simulink model "LQG_tw_v2"  (R2019a)
settings: Solver=FixedStepAuto  StartTime=0.0  StopTime=15  FixedStep=0.01  RelTol=1e-3
undefined symbols (not defined in the file): AA, BB, C, K, L
libraries: simulink x2, simulink_extras x1
settings Model: Creator=chute  LastModifiedBy=chute
settings DataIOCC: ReturnWorkspaceOutputs=off

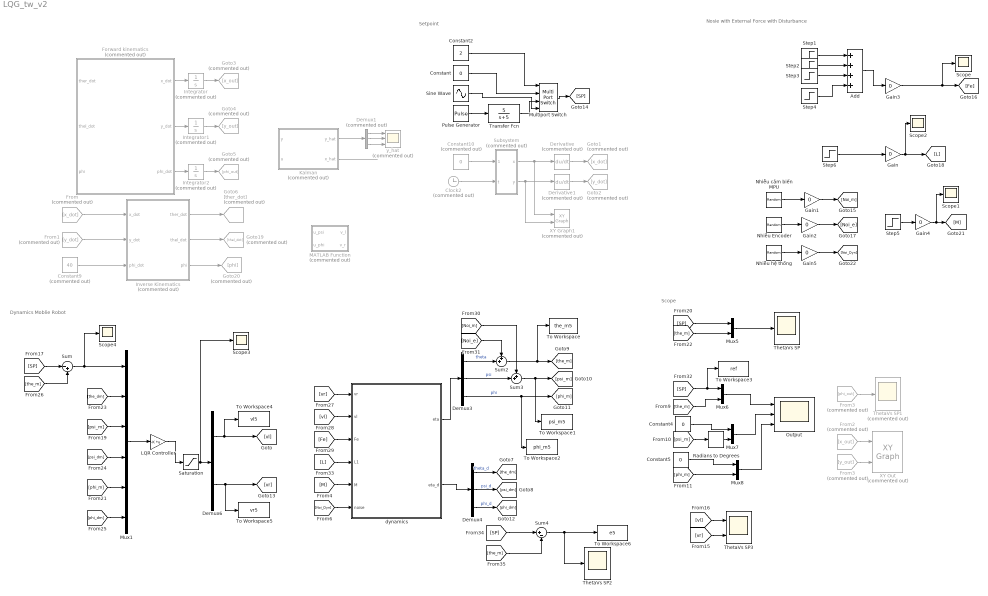
== system LQG_tw_v2 ==
  note: Nosie with External Force with Disturbance
  note: Scope
  note: Setpoint
  note: Dynamics Moblie Robot
  Add : Sum  Inputs=++++
  Clock2 : Clock  Commented=on
  Constant : Constant  Value=0
  Constant10 : Constant  Commented=on  Value=0
  Constant2 : Constant  Value=2
  Constant4 : Constant  Value=0
  Constant5 : Constant  Value=0
  Constant9 : Constant  Commented=on  Value=40
  Demux1 : Demux  Commented=on  Outputs=3
  Demux3 : Demux  Outputs=3
  Demux4 : Demux  Outputs=3
  Demux6 : Demux  Outputs=2
  Derivative : Derivative  Commented=on
  Derivative1 : Derivative  Commented=on
  Forward kinematics : MATLAB Function  Commented=on  TreatAsAtomicUnit=on
  From : From  Commented=on  GotoTag=x_dot
  From1 : From  Commented=on  GotoTag=y_dot
  From2 : From  Commented=on  GotoTag=x_out
  From3 : From  Commented=on  GotoTag=phi_out
  "From3 " : From  Commented=on  GotoTag=y_out
  Gain{,1..5} (6 alike) : Gain  Gain=0
  Goto1 : Goto  Commented=on  GotoTag=x_dot
  Goto19 : Goto  Commented=on  GotoTag=thel_dot
  Goto2 : Goto  Commented=on  GotoTag=y_dot
  Goto20 : Goto  Commented=on  GotoTag=phi
  Goto3 : Goto  Commented=on  GotoTag=x_out
  Goto4 : Goto  Commented=on  GotoTag=y_out
  Goto5 : Goto  Commented=on  GotoTag=phi_out
  Goto6 : Goto  Commented=on  GotoTag=ther_dot
  Integrator : Integrator  Commented=on
  Integrator1 : Integrator  Commented=on
  Integrator2 : Integrator  Commented=on  InitialCondition=[0;0]
  Inverse Kinematics : MATLAB Function  Commented=on  TreatAsAtomicUnit=on
  Kalman : Subsystem  Commented=on
  LQR Controller : Gain  Gain=-K  Multiplication=Matrix(K*u) (u vector)
  MATLAB Function : MATLAB Function  Commented=on  TreatAsAtomicUnit=on
  Multiport Switch : MultiPortSwitch
  Mux1 : Mux  Inputs=6
  Mux{5..8} (4 alike) : Mux  Inputs=2
  Nhiễu Encoder : RandomNumber  Variance=0.0001  SampleTime=0.01
  Nhiễu cảm biến MPU : RandomNumber  Variance=0.0005  SampleTime=0.01
  Nhiễu hệ thống : RandomNumber  Variance=0.0001  SampleTime=0.01
  Output : Scope  NumInputPorts=3
  Pulse Generator : DiscretePulseGenerator  PulseType=Time based  Amplitude=3.14  Period=10  PulseWidth=50
  Radians to Degrees : simulink_extras/Transformations/Radians to Degrees
  Saturation : Saturate  UpperLimit=12  LowerLimit=-12
  Scope{,1..4} (5 alike) : Scope
  Sine Wave : Sin  Amplitude=3.14  Frequency=0.1*pi  SampleTime=0
  Step1 : Step  Time=3  After=0.3  SampleTime=0
  Step2 : Step  Time=4  After=-0.3  SampleTime=0
  Step3 : Step  Time=10  After=0.3  SampleTime=0
  Step4 : Step  Time=11  After=-0.3  SampleTime=0
  Step5 : Step  Time=8  Before=0.945  After=1000  SampleTime=0
  Step6 : Step  Time=5  Before=0.121/2  After=0.121/2+0.1  SampleTime=0
  Subsystem : Subsystem  Commented=on
  Sum : Sum  Inputs=|-+
  Sum2 : Sum  Inputs=++|
  Sum3 : Sum  Inputs=++|
  Sum4 : Sum  Inputs=|+-
  ThetaVs SP : Scope
  ThetaVs SP1 : Scope  Commented=on
  ThetaVs SP2 : Scope
  ThetaVs SP3 : Scope  NumInputPorts=2
  To Workspace : ToWorkspace  VariableName=the_m5  SaveFormat=Structure With Time  SampleTime=-1
  To Workspace1 : ToWorkspace  VariableName=psi_m5  SaveFormat=Structure With Time  SampleTime=-1
  To Workspace2 : ToWorkspace  VariableName=phi_m5  SaveFormat=Structure With Time  SampleTime=-1
  To Workspace3 : ToWorkspace  VariableName=ref  SaveFormat=Structure With Time  SampleTime=-1
  To Workspace4 : ToWorkspace  VariableName=vl5  SaveFormat=Structure With Time  SampleTime=-1
  To Workspace5 : ToWorkspace  VariableName=vr5  SaveFormat=Structure With Time  SampleTime=-1
  To Workspace6 : ToWorkspace  VariableName=e5  SaveFormat=Structure With Time  SampleTime=-1
  Transfer Fcn : TransferFcn  Numerator=[5]  Denominator="[1  5]"
  XY Graph1 : simulink/Sinks/XY Graph  Commented=on  xmin=-1  xmax=1  ymin=-1  ymax=1  st=-1
  XY Out : simulink/Sinks/XY Graph  Commented=on  xmin=-1  xmax=1  ymin=-1  ymax=1  st=-1
  dynamics : Subsystem
  y_hat : Scope  Commented=on  NumInputPorts=3
  wires:
  dynamics/1(eta) -> Demux3/1
  Demux4/1 -> [the_dm]  "theta_d"
  dynamics/2(eta_d) -> Demux4/1
  Demux4/3 -> [phi_dm]  "phi_d"
  Demux4/2 -> [psi_dm]  "psi_d"
  Demux6/1 -> To Workspace4/1, [vl]
  LQR Controller/1 -> Saturation/1
  Mux1/1 -> LQR Controller/1
  Sum/1 -> Scope4/1, Mux1/1
  Multiport Switch/1 -> [SP]
  Constant/1 -> Multiport Switch/2
  Constant2/1 -> Multiport Switch/1
  Mux5/1 -> ThetaVs SP/1
  [SP] -> Mux5/1
  [the_m] -> Mux5/2
  [phi_m] -> Mux1/5
  [psi_m] -> Mux1/3
  [the_dm] -> Mux1/2
  [psi_dm] -> Mux1/4
  [phi_dm] -> Mux1/6
  Nhiễu cảm biến MPU/1 -> Gain1/1
  Demux3/3 -> To Workspace2/1, [phi_m]  "phi"
  Sum3/1 -> To Workspace1/1, [psi_m]
  Demux3/2 -> Sum3/2  "psi"
  Demux3/1 -> Sum2/2  "theta"
  Nhiễu Encoder/1 -> Gain2/1
  [the_m] -> Sum/2
  Sine Wave/1 -> Multiport Switch/4
  [vl] -> dynamics/2("vl ")
  [vr] -> dynamics/1(vr)
  [Fe] -> dynamics/3(Fe)
  Gain1/1 -> [Noi_m]
  Gain2/1 -> [Noi_e]
  [Noi_m] -> Sum3/1
  [Noi_e] -> Sum2/1
  Add/1 -> Gain3/1
  Mux8/1 -> Output/3
  Mux7/1 -> Output/2
  Mux6/1 -> Output/1
  [the_m] -> Mux6/2
  [SP] -> To Workspace3/1, Mux6/1
  [psi_m] -> Radians to Degrees/1
  Constant4/1 -> Mux7/1
  [phi_m] -> Mux8/2
  Constant5/1 -> Mux8/1
  [L] -> dynamics/4(L1)
  Step6/1 -> Gain/1
  Gain/1 -> Scope2/1, [L]
  Sum2/1 -> To Workspace/1, [the_m]
  Demux6/2 -> To Workspace5/1, [vr]
  [SP] -> Sum4/1
  [the_m] -> Sum4/2
  Sum4/1 -> ThetaVs SP2/1, To Workspace6/1
  Pulse Generator/1 -> Transfer Fcn/1
  [SP] -> Sum/1
  Transfer Fcn/1 -> Multiport Switch/3
  Forward kinematics/1(x_dot) -> Integrator/1
  Forward kinematics/3(phi_dot) -> Integrator2/1
  Clock2/1 -> Subsystem/2(t)
  Subsystem/1(x) -> Derivative/1, XY Graph1/1
  Constant10/1 -> Subsystem/1(mode)
  Forward kinematics/2(y_dot) -> Integrator1/1
  Constant9/1 -> Inverse Kinematics/3(phi_dot)
  Integrator2/1 -> Goto5/1
  Subsystem/2(y) -> XY Graph1/2, Derivative1/1
  Derivative1/1 -> Goto2/1
  Derivative/1 -> Goto1/1
  From1/1 -> Inverse Kinematics/2(y_dot)
  From/1 -> Inverse Kinematics/1(x_dot)
  Integrator/1 -> Goto3/1
  Integrator1/1 -> Goto4/1
  From2/1 -> XY Out/1
  "From3 "/1 -> XY Out/2
  From3/1 -> ThetaVs SP1/1
  Inverse Kinematics/1(ther_dot) -> Goto6/1
  Inverse Kinematics/2(thel_dot) -> Goto19/1
  Inverse Kinematics/3(phi) -> Goto20/1
  Kalman/1(y_hat) -> Demux1/1
  Demux1/1 -> y_hat/1
  Demux1/3 -> y_hat/3
  Demux1/2 -> y_hat/2
  Kalman/2(x_hat) -> ?
  Step1/1 -> Add/1
  Step2/1 -> Add/2
  Gain3/1 -> Scope/1, [Fe]
  Step4/1 -> Add/4
  Step3/1 -> Add/3
  Step5/1 -> Gain4/1
  Gain4/1 -> Scope1/1, [M]
  [M] -> dynamics/5(M)
  Gain5/1 -> [Noi_Dyn]
  Nhiễu hệ thống/1 -> Gain5/1
  [Noi_Dyn] -> dynamics/6(noise)
  Saturation/1 -> Scope3/1, Demux6/1
  Radians to Degrees/1 -> Mux7/2
  [vl] -> ThetaVs SP3/1
  [vr] -> ThetaVs SP3/2

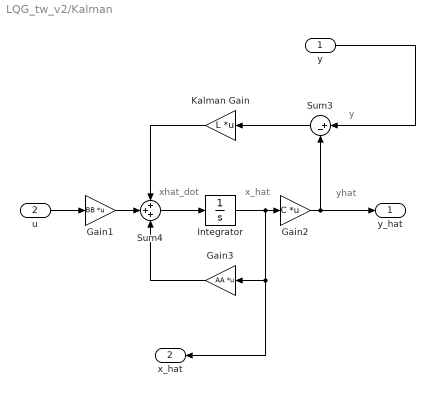
== system LQG_tw_v2/Kalman ==
  note: x_hat
  note: yhat
  note: xhat_dot
  note: y
  y : Inport
  u : Inport  Port=2
  Gain1 : Gain  Gain=BB  Multiplication=Matrix(K*u)
  Gain2 : Gain  Gain=C  Multiplication=Matrix(K*u)
  Gain3 : Gain  Gain=AA  Multiplication=Matrix(K*u)
  Integrator : Integrator  InitialCondition=[0.5;0.01;pi/6;0.001;0.0;0.001]
  Kalman Gain : Gain  Gain=L  Multiplication=Matrix(K*u)
  Sum3 : Sum  Inputs=|+-
  Sum4 : Sum  Inputs=+++
  y_hat : Outport
  x_hat : Outport  Port=2
  wires:
  u/1 -> Gain1/1
  Integrator/1 -> x_hat/1, Gain3/1, Gain2/1
  Gain1/1 -> Sum4/2
  Gain2/1 -> y_hat/1, Sum3/2
  Sum4/1 -> Integrator/1
  y/1 -> Sum3/1
  Gain3/1 -> Sum4/3
  Kalman Gain/1 -> Sum4/1
  Sum3/1 -> Kalman Gain/1

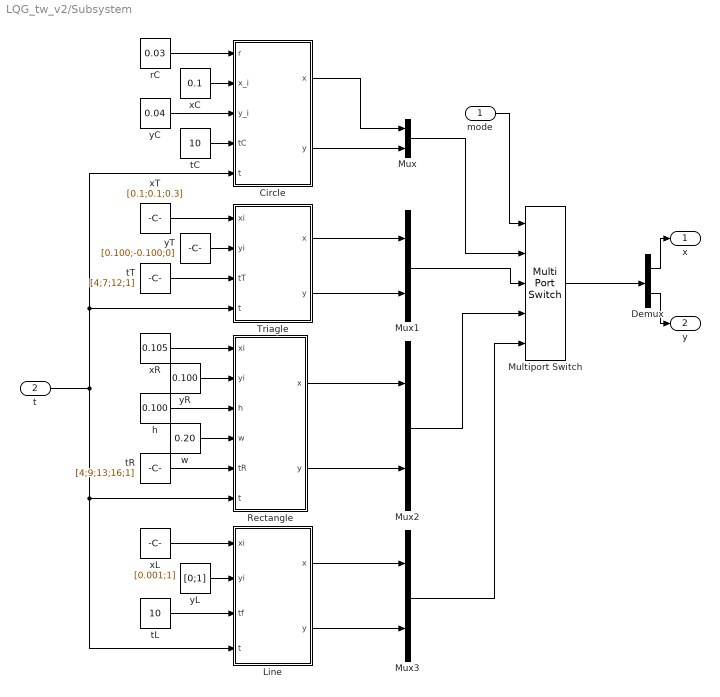
== system LQG_tw_v2/Subsystem ==
  mode : Inport
  t : Inport  Port=2
  Circle : MATLAB Function  TreatAsAtomicUnit=on
  Demux : Demux  Outputs=2
  Line : MATLAB Function  TreatAsAtomicUnit=on
  Multiport Switch : MultiPortSwitch  DataPortOrder=Zero-based contiguous  Inputs=4  zeroidx=on
  Mux{,1..3} (4 alike) : Mux  Inputs=2
  Rectangle : MATLAB Function  TreatAsAtomicUnit=on
  Triagle : MATLAB Function  TreatAsAtomicUnit=on
  h : Constant  Value=0.100
  rC : Constant  Value=0.03
  tC : Constant  Value=10
  tL : Constant  Value=10
  tR : Constant  Value=[4;9;13;16;1]
  tT : Constant  Value=[4;7;12;1]
  w : Constant  Value=0.20
  xC : Constant  Value=0.1
  xL : Constant  Value=[0.001;1]
  xR : Constant  Value=0.105
  xT : Constant  Value=[0.1;0.1;0.3]
  yC : Constant  Value=0.04
  yL : Constant  Value=[0;1]
  yR : Constant  Value=0.100
  yT : Constant  Value=[0.100;-0.100;0]
  x : Outport
  y : Outport  Port=2
  wires:
  tR/1 -> Rectangle/5(tR)
  xL/1 -> Line/1(xi)
  Line/1(x) -> Mux3/1
  tC/1 -> Circle/4(tC)
  yL/1 -> Line/2(yi)
  tT/1 -> Triagle/3(tT)
  Multiport Switch/1 -> Demux/1
  Line/2(y) -> Mux3/2
  Triagle/1(x) -> Mux1/1
  Mux3/1 -> Multiport Switch/5
  xR/1 -> Rectangle/1(xi)
  Circle/2(y) -> Mux/2
  tL/1 -> Line/3(tf)
  w/1 -> Rectangle/4(w)
  Mux2/1 -> Multiport Switch/4
  mode/1 -> Multiport Switch/1
  Circle/1(x) -> Mux/1
  Mux1/1 -> Multiport Switch/3
  rC/1 -> Circle/1(r)
  Mux/1 -> Multiport Switch/2
  h/1 -> Rectangle/3(h)
  t/1 -> Circle/5(t), Triagle/4(t), Rectangle/6(t), Line/4(t)
  Demux/1 -> x/1
  xT/1 -> Triagle/1(xi)
  Rectangle/1(x) -> Mux2/1
  yT/1 -> Triagle/2(yi)
  xC/1 -> Circle/2(x_i)
  Triagle/2(y) -> Mux1/2
  yR/1 -> Rectangle/2(yi)
  Demux/2 -> y/1
  Rectangle/2(y) -> Mux2/2
  yC/1 -> Circle/3(y_i)

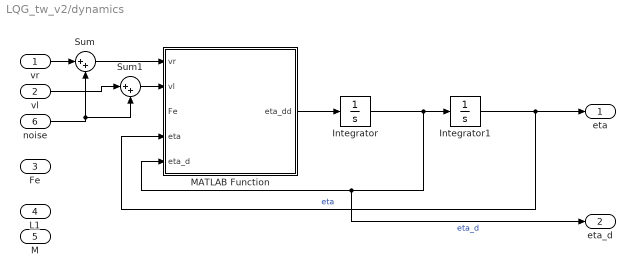
== system LQG_tw_v2/dynamics ==
  vr : Inport
  "vl " : Inport  Port=2
  Fe : Inport  Port=3
  L1 : Inport  Port=4
  M : Inport  Port=5
  noise : Inport  Port=6
  Integrator : Integrator  InitialCondition=[0;0;0]
  Integrator1 : Integrator  InitialCondition=[0;0.3*pi/180;0]
  MATLAB Function : MATLAB Function  TreatAsAtomicUnit=on
  Sum : Sum  Inputs=|++
  Sum1 : Sum  Inputs=|++
  eta : Outport
  eta_d : Outport  Port=2
  wires:
  Integrator/1 -> Integrator1/1, eta_d/1, MATLAB Function/5(eta_d)  "eta_d"
  Integrator1/1 -> eta/1, MATLAB Function/4(eta)  "eta"
  MATLAB Function/1(eta_dd) -> Integrator/1
  vr/1 -> Sum/1
  Sum/1 -> MATLAB Function/1(vr)
  Sum1/1 -> MATLAB Function/2(vl)
  "vl "/1 -> Sum1/1
  noise/1 -> Sum1/2, Sum/2

== matlab function LQG_tw_v2/Forward kinematics ==
  data: ther_dot input; x_dot output; thel_dot input; y_dot output; phi_dot output; phi input
function [x_dot,y_dot,phi_dot] = FK(ther_dot,thel_dot,phi)
R =0.0335; % Wheel radius
W =0.17; % Body width
% thel_dot= (the_dot-(phi_dot*W)/R);
% ther_dot= the_dot+phi_dot*W/(2*R);
for i=1:2
    J=[(R/2)*cos(phi(i)),(R/2)*cos(phi(i));
        (R/2)*sin(phi(i)),(R/2)*sin(phi(i));
        R/W,-R/W];
end
out =J*[ther_dot;thel_dot];
x_dot=out(1,1);
y_dot =out(2,1);
phi_dot =out(3,1);


end

== matlab function LQG_tw_v2/dynamics/MATLAB Function ==
  data: vr input; vl input; Fe input; eta_dd output; eta input; eta_d input
function eta_dd= fcn(vr,vl,Fe,eta,eta_d)
%% declare the parameter:
%% Hoang

g =9.81; % gravity acceleration
m =0.046; % wheel weight
R =0.0335; % Wheel radius
M =0.945;  % body weight
W =0.17; % Body width
D =0.1; % Body depth
H =0.121;% Body Height
L =0.121/2;% distance

n =30 ; %gear ratio
Rm=8.0013;      %dien tro dong co DC
Kb=0.45096;   %he so emf cua dong co
Kt=0.45096;   %momemt xoan cua dong co DC\
fm = 0.21895; % friction cof between body and DC motor.
fw = 0.01; % friction cof between wheel and floor
anp = (n*Kt)/Rm;
bet = (n*Kt*Kb/Rm)+fm;

J_psi  = M*L^2/3; % Body inertia moment
Jw = m*R^2/2;  %Wheel inertia moment
J_phi = M*(W^2+D^2)/12; % Body yaw inertia moment
Jm = 0.00083134;
anp = (n*Kt)/Rm;
bet = (n*Kt*Kb/Rm)+fm;

%% Notation:
the=eta(1,1);
psi=eta(2,1);
phi=eta(3,1);

the_dot=eta_d(1,1);
psi_dot=eta_d(2,1);
phi_dot=eta_d(3,1);

tor=[vl;vr];



%% DC Motor
F_the = anp*(vl+vr)-2*(bet+fw)*the_dot+2*bet*psi_dot;
F_psi = -anp*(vl+vr)+2*bet*the_dot-2*bet*psi_dot;
F_phi = W*anp*(vr-vl)/(2*R)-W^2*((bet+fw)*phi_dot)/2*R^2;
tor =[F_the;F_psi;F_phi];

%% dyn
% Mass matrix:
M1 = ...
[2*Jw + 2*Jm*n^2 + R^2*(M + 2*m),L*M*R*cos(psi) - 2*Jm*n^2,0;
 L*M*R*cos(psi) - 2*Jm*n^2,J_psi + L^2*M + 2*Jm*n^2,0;
 0,0,J_phi + (W^2*m)/2 + L^2*M*sin(psi)^2 + (W^2*(Jw + Jm*n^2))/(2*R^2)];

%Coriolis matrix:
C1 = ...
[0,-L*M*R*psi_dot*sin(psi),0;
 0,0,-(L^2*M*phi_dot*sin(2*psi))/2;
 0,(L^2*M*phi_dot*sin(2*psi))/2,(L^2*M*psi_dot*sin(2*psi))/2];


% Gravity vector:
G1=...
[0;
-L*M*g*sin(psi);
0];
%% Input Matrices:
% B1=[1/R,        1/R;
%     -1,          -1;
%     W/(2*R),-W/(2*R)];

%% External Force
Fe=[0;Fe;0];

eta_dd=inv(M1)*(tor-C1*eta_d-G1);
end

== matlab function LQG_tw_v2/MATLAB Function ==
  data: u_psi input; v_l output; u_phi input; v_r output
function [v_l,v_r] = fcn(u_psi,u_phi)
v_l=(1/2)*(u_psi-u_phi);
v_r=(1/2)*(u_psi+u_phi);

end

== matlab function LQG_tw_v2/Inverse Kinematics ==
  data: x_dot input; ther_dot output; y_dot input; phi_dot input; thel_dot output; phi output
function [ther_dot,thel_dot,phi] = fcn(x_dot,y_dot,phi_dot)

R =0.0335; % Wheel radius
W =0.17; % Body width
a=y_dot;
b=-x_dot;
d=0;
anp = atan2(b, a);
x1 = anp + atan2(sqrt(a*a + b*b - d*d), d);
x2 = anp + atan2(-sqrt(a*a + b*b - d*d), d);
phi=[x1;x2];
    for i=1:2
        j=[cos(phi(i))/R,sin(phi(i))/R,W/(2*R);
           cos(phi(i))/R,sin(phi(i))/R,-W/(2*R)];
        out1=j*[x_dot;y_dot;phi_dot];
    end
ther_dot=out1(1,1);
thel_dot=out1(2,1);

== matlab function LQG_tw_v2/Subsystem/Circle ==
  data: x output; r input; x_i input; y_i input; tC input; y output; t input
% Circle
function [x,y] = fcn(r,x_i,y_i,tC,t)
t0 = 3;
if (t-t0) <=tC
    x = x_i + r*cos(2*pi*(t-t0)/tC);
    y = y_i + r*sin(2*pi*(t-t0)/tC);
else
    x = x_i + r*cos(2*pi);
    y = y_i + r*sin(2*pi);
end

== matlab function LQG_tw_v2/Subsystem/Line ==
  data: x output; xi input; yi input; tf input; y output; t input
% Triangle
function [x,y] = fcn(xi,yi,tf,t)
A = [xi(1);yi(1)];
B = [xi(2);yi(2)];
v0 = [0;0];
vf = [0;0];
t0=0;
if t<=tf
    Y = transpose([A v0 B vf]);
    K = [1 t0 t0^2 t0^3;
         0  1 2*t0 3*t0^2;
         1 tf tf^2 tf^3;
         0  1 2*tf 3*tf^2];
    X = inv(K)*Y;
    a = transpose(X);
    x = a(1,1) + a(1,2)*t + a(1,3)*t^2 + a(1,4)*t^3;

    y = a(2,1) + a(2,2)*t + a(2,3)*t^2 + a(2,4)*t^3;
else
    x = B(1);
    y = B(2);
end

== matlab function LQG_tw_v2/Subsystem/Rectangle ==
  data: x output; xi input; yi input; h input; w input; tR input; y output; t input
% rectangle
function [x,y] = fcn(xi,yi,h,w,tR,t)
x1 = xi;
x2 = xi + w;
x3 = x2;
x4 = x1;
y1 = yi;
y2 = y1;
y3 = yi - h;
y4 = y3;
A = [x1;y1];
B = [x2;y2];
C = [x3;y3];
D = [x4;y4];
v0 = [0;0];
vf = [0;0];
t0=0;t1=tR(1);t2=tR(2);t3=tR(3);tf=tR(4);
td = tR(5);
td1 = t1+td;
td2 = t2+td;
td3 = t3+td;
if t<=t1
    Y = transpose([A v0 B vf]);
    K = [1 t0 t0^2 t0^3;
         0  1 2*t0 3*t0^2;
         1 t1 t1^2 t1^3;
         0  1 2*t1 3*t1^2];
    X = inv(K)*Y;
    a = transpose(X);
    x = a(1,1) + a(1,2)*t + a(1,3)*t^2 + a(1,4)*t^3;

    y = a(2,1) + a(2,2)*t + a(2,3)*t^2 + a(2,4)*t^3;
elseif (t>t1) && (t<=td1)
    x = B(1);y = B(2);
elseif (t>td1) && (t<=t2)
    Y = transpose([B v0 C vf]);
    K = [1 td1 td1^2 td1^3;
         0  1 2*td1 3*td1^2;
         1 t2 t2^2 t2^3;
         0  1 2*t2 3*t2^2];
    X = inv(K)*Y;
    a = transpose(X);
    x = a(1,1) + a(1,2)*t + a(1,3)*t^2 + a(1,4)*t^3;

    y = a(2,1) + a(2,2)*t + a(2,3)*t^2 + a(2,4)*t^3;
elseif (t>t2) && (t<=td2)
    x = C(1);y = C(2);
elseif (t>td2) && (t<=t3)
    Y = transpose([C v0 D vf]);
    K = [1 td2 td2^2 td2^3;
         0  1 2*td2 3*td2^2;
         1 t3 t3^2 t3^3;
         0  1 2*t3 3*t3^2];
    X = inv(K)*Y;
    a = transpose(X);
    x = a(1,1) + a(1,2)*t + a(1,3)*t^2 + a(1,4)*t^3;

    y = a(2,1) + a(2,2)*t + a(2,3)*t^2 + a(2,4)*t^3;
elseif (t>t3) && (t<=td3)
    x = D(1);y = D(2);
elseif (t>td3) && (t<=tf)
    Y = transpose([D v0 A vf]);
    K = [1 td3 td3^2 td3^3;
         0  1 2*td3 3*td3^2;
         1 tf tf^2 tf^3;
         0  1 2*tf 3*tf^2];
    X = inv(K)*Y;
    a = transpose(X);
    x = a(1,1) + a(1,2)*t + a(1,3)*t^2 + a(1,4)*t^3;

    y = a(2,1) + a(2,2)*t + a(2,3)*t^2 + a(2,4)*t^3;
else
    x = A(1);
    y = A(2);
end

== matlab function LQG_tw_v2/Subsystem/Triagle ==
  data: x output; xi input; yi input; tT input; y output; t input
% Triangle
function [x,y] = fcn(xi,yi,tT,t)
A = [xi(1);yi(1)];
B = [xi(2);yi(2)];
C = [xi(3);yi(3)];
v0 = [0;0];
vf = [0;0];
t0=0;t1=tT(1);t2=tT(2);tf=tT(3);td = tT(1) + tT(4); tdd = tT(2) + tT(4);
if t<=t1
    Y = transpose([A v0 B vf]);
    K = [1 t0 t0^2 t0^3;
         0  1 2*t0 3*t0^2;
         1 t1 t1^2 t1^3;
         0  1 2*t1 3*t1^2];
    X = inv(K)*Y;
    a = transpose(X);
    x = a(1,1) + a(1,2)*t + a(1,3)*t^2 + a(1,4)*t^3;

    y = a(2,1) + a(2,2)*t + a(2,3)*t^2 + a(2,4)*t^3;
elseif (t>t1) && (t<=td)
    x = B(1);y = B(2);
elseif (t>td) && (t<=t2)
    Y = transpose([B v0 C vf]);
    K = [1 td td^2 td^3;
         0  1 2*td 3*td^2;
         1 t2 t2^2 t2^3;
         0  1 2*t2 3*t2^2];
    X = inv(K)*Y;
    a = transpose(X);
    x = a(1,1) + a(1,2)*t + a(1,3)*t^2 + a(1,4)*t^3;

    y = a(2,1) + a(2,2)*t + a(2,3)*t^2 + a(2,4)*t^3;
elseif (t>t2) && (t<=tdd)
    x = C(1);y = C(2);
elseif (t>tdd) && (t<=tf)
    Y = transpose([C v0 A vf]);
    K = [1 tdd tdd^2 tdd^3;
         0  1 2*tdd 3*tdd^2;
         1 tf tf^2 tf^3;
         0  1 2*tf 3*tf^2];
    X = inv(K)*Y;
    a = transpose(X);
    x = a(1,1) + a(1,2)*t + a(1,3)*t^2 + a(1,4)*t^3;

    y = a(2,1) + a(2,2)*t + a(2,3)*t^2 + a(2,4)*t^3;
else
    x = A(1);y = A(2);
end
